simulink subsystem "DeserializeUINT16"  (R2019b)
settings: Solver=VariableStepAuto  StartTime=0.0  StopTime=10.0  RelTol=1e-3
settings Model: Creator=VM  LastModifiedBy=VM

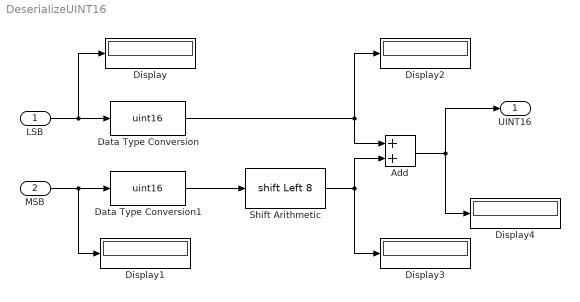
== system DeserializeUINT16 ==
  LSB : Inport  OutDataTypeStr=uint8
  MSB : Inport  Port=2  OutDataTypeStr=uint8
  Add : Sum
  Data Type Conversion : DataTypeConversion  OutDataTypeStr=uint16
  Data Type Conversion1 : DataTypeConversion  OutDataTypeStr=uint16
  Display{,1..4} (5 alike) : Display
  Shift Arithmetic : ArithShift  BitShiftNumber=8  BitShiftDirection=Left
  UINT16 : Outport  OutDataTypeStr=uint16  LockScale=on
  wires:
  Data Type Conversion1/1 -> Shift Arithmetic/1
  MSB/1 -> Data Type Conversion1/1, Display1/1
  Add/1 -> UINT16/1, Display4/1
  Data Type Conversion/1 -> Add/1, Display2/1
  Shift Arithmetic/1 -> Add/2, Display3/1
  LSB/1 -> Data Type Conversion/1, Display/1
